simulink model "RF_KC_Time_AxisA4"  (R2020a)
settings: Solver=FixedStepAuto  StartTime=0.0  StopTime=10  FixedStep=0.001  RelTol=1e-3  EnableMultiTasking=on
values from neighbouring files (symbols this model uses):
  A_DC_ESO = [-L1 1 0 0;-L2 0 1 0;-L3 0 0 0;0 0 L4_DCESO/b0 0;]    [Code2.m]
  A_ESO = [-L1 1 0;-L2 0 1;-L3 0 0]    [Code2.m]
  A_ESO2 = [-L1 1 0;-L2 0 1;-L3 0 0]    [Code2.m]
  A_GPIO = [-L1 1 0 0;-L2 0 1 0;-L3 0 0 1; -L4 0 0 0]    [Code2.m]
  b0 = 80    [Code2.m]
  B_DC_ESO = [0 L1;b0 L2;0 L3;0 0]    [Code2.m]
  B_ESO = [0 L1;b0 L2;0 L3]    [Code2.m]
  B_ESO2 = [0 L1;b0 L2;0 L3]    [Code2.m]
  B_GPIO = [0 L1;b0 L2;0 L3;0 L4]    [Code2.m]
  C_DC_ESO = eye(4)    [Code2.m]
  C_ESO = eye(3)    [Code2.m]
  C_ESO2 = eye(3)    [Code2.m]
  C_GPIO = eye(4)    [Code2.m]
  D_DC_ESO = [0 0;0 0;0 0;0 0]    [Code2.m]
  D_ESO = [0 0;0 0;0 0]    [Code2.m]
  D_ESO2 = [0 0;0 0;0 0]    [Code2.m]
  D_GPIO = [0 0;0 0;0 0;0 0]    [Code2.m]
  den_G_invse = den_G_invse{1,1}    [Code2.m]
  den_Q = den_Q{1,1}    [Code2.m]
  num_G_invse = num_G_invse{1,1}    [Code2.m]
  num_Q = num_Q{1,1}    [Code2.m]
  wc = 3*2*pi    (= 18.8495559215)    [Code2.m]
undefined symbols (not defined in the file or in its folder): den_GV, num_GV, taoP
libraries: simulink x1, commnoisgen2 x1
settings Model: Creator=chaosir  LastModifiedBy=Laptop
settings DataIOCC: LimitDataPoints=on  SaveFormat=StructureWithTime  ReturnWorkspaceOutputs=off
settings OptimizationCC: LifeSpan=inf
settings DebuggingCC: SolverPrmCheckMsg=warning  SFUnexpectedBacktrackingDiag=warning  SFNoUnconditionalDefaultTransitionDiag=warning  SFExecutionAtInitializationDiag=none  ArithmeticOperatorsInVariantConditions=warning
settings HardwareCC: ProdBitPerPointer=32  ProdBitPerSizeT=32  ProdBitPerPtrDiffT=32  ProdLargestAtomicFloat=None  ProdIntDivRoundTo=Undefined  ProdEndianess=Unspecified  ProdWordSize=32  ProdHWDeviceType=32-bit Generic
settings ModelReferenceCC: PropagateSignalLabelsOutOfModel=off
settings SFSimCC: SimUseLocalCustomCode=off  CustomCodeUndefinedFunction=UseInterfaceOnly
settings RTWCC: RTWUseLocalCustomCode=off
settings CodeAppCC: StateflowObjectComments=on
settings GRTTargetCC: TargetLangStandard=C89/C90 (ANSI)
settings ConfigComp: CovMetricSettings=dw  CovHtmlReporting=on  CovSaveCumulativeToWorkspaceVar=on  CovSaveSingleToWorkspaceVar=on  CovExternalEMLEnable=off  CovSFcnEnable=off
settings SimscapeCC: SimscapeNormalizeSystem=off
settings ConfigurationSet: Description=SimMechanics 2G

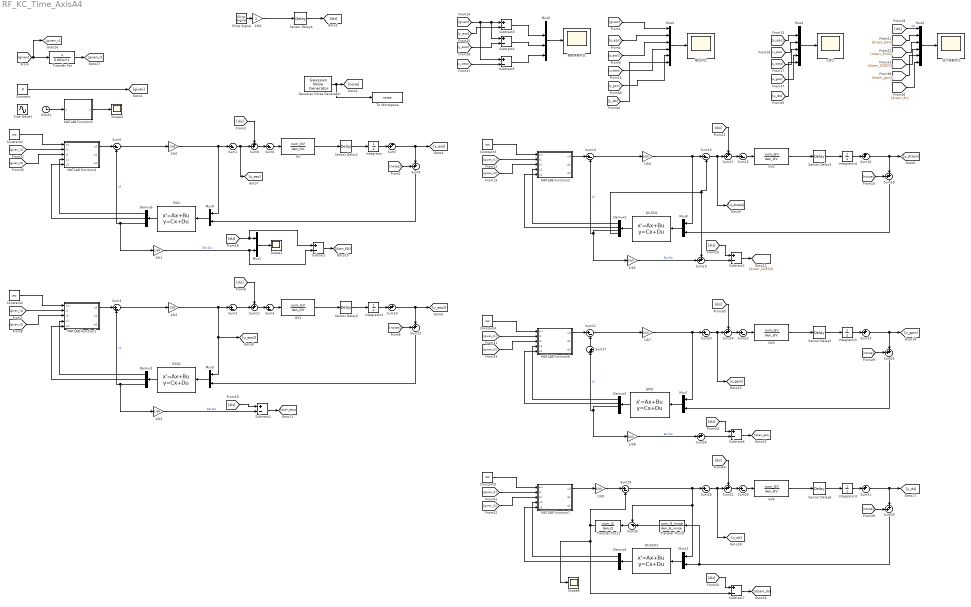
== system RF_KC_Time_AxisA4 ==
  1/b{0..5,7..9} (9 alike) : Gain  Gain=1/b0
  1/b6 : Gain  Gain=2
  Chirp Signal : simulink/Sources/Chirp Signal  f1=0.2  T=7.5  f2=1
  Clock1 : Clock
  Constant : Constant  Value=0
  Constant{1..5} (5 alike) : Constant  Value=wc
  DC-ESO : StateSpace  A=A_DC_ESO  B=B_DC_ESO  C=C_DC_ESO  D=D_DC_ESO
  DC-ESO1 : StateSpace  A=A_ESO  B=B_ESO  C=C_ESO  D=D_ESO
  Demux1 : Demux  Outputs=3
  Demux2 : Demux
  Demux3 : Demux
  Demux4 : Demux  Outputs=3
  Demux5 : Demux  Outputs=3
  ESO : StateSpace  A=A_ESO  B=B_ESO  C=C_ESO  D=D_ESO
  ESO2 : StateSpace  A=A_ESO2  B=B_ESO2  C=C_ESO2  D=D_ESO2
  GPIO : StateSpace  A=A_GPIO  B=B_GPIO  C=C_GPIO  D=D_GPIO
  GV{,1..4} (5 alike) : TransferFcn  Numerator=num_GV  Denominator=den_GV
  Gaussian Noise Generator : commnoisgen2/Gaussian Noise Generator  m=0  d=1e-6  s=0  Ts=0.001  frameBased=off  sampPerFrame=1  orient=off  outDataType=double
      settings: SourceProductBaseCode=CM
  Integrator{,1..4} (5 alike) : Integrator
  MATLAB Function1 : MATLAB Function  TreatAsAtomicUnit=on
  MATLAB Function2 : MATLAB Function  TreatAsAtomicUnit=on
  MATLAB Function4 : MATLAB Function  TreatAsAtomicUnit=on
  MATLAB Function5 : MATLAB Function  TreatAsAtomicUnit=on
  MATLAB Function6 : MATLAB Function  TreatAsAtomicUnit=on
  MATLAB Function7 : MATLAB Function  TreatAsAtomicUnit=on
  Mux{1,5,7..9,11} (6 alike) : Mux  Inputs=2
  Mux2 : Mux  Inputs=6
  Mux3 : Mux  Inputs=6
  Mux4 : Mux  Inputs=6
  Mux6 : Mux
  Scope1 : Scope
  Scope3 : Scope
  Scope6 : Scope
  Sensor Delay{1..3,5..6} (5 alike) : TransportDelay  DelayTime=taoP  PadeOrder=5
  Sensor Delay4 : TransportDelay  DelayTime=3  PadeOrder=5
  Sine Wave1 : Sin  Amplitude=40  Frequency=2*pi*0.08  SampleTime=0
  Subtract{,1..7} (8 alike) : Sum  Inputs=+-
  Sum{1..6,13..15,20..22,28..30} (15 alike) : Sum  Inputs=|+-
  Sum{7..12,16..19,23..26,31..33} (17 alike) : Sum  Inputs=++|
  Sum27 : Sum  Inputs=|++
  Sum35 : Sum  Inputs=-+|
  To Workspace : ToWorkspace  VariableName=noise  SampleTime=-1
  Transfer Fcn : TransferFcn  Numerator=[1 0]  Denominator=[0.001 1]
  Transfer Fcn10 : TransferFcn  Numerator=num_G_invse  Denominator=den_G_invse
  Transfer Fcn11 : TransferFcn  Numerator=num_Q  Denominator=den_Q
  u对比 : Scope
  估计误差对比 : Scope
  跟踪误差对比 : Scope
  输出对比 : Scope
  wires:
  Mux9/1 -> ESO/1
  ESO/1 -> Demux5/1
  Sum1/1 -> [u_eso], Sum8/2
  Mux2/1 -> 输出对比/1
  Sum6/1 -> GV/1
  Demux5/3 -> Sum5/2, 1/b1/1  "z3"
  Sum5/1 -> 1/b0/1
  Sensor Delay1/1 -> Integrator/1
  Sum9/1 -> Mux9/2
  Integrator/1 -> Sum7/2
  Sum8/1 -> Sum6/1
  [noise] -> Sum9/1
  Sum7/1 -> Sum9/2, [y_eso]
  Constant1/1 -> MATLAB Function4/1(wc)
  Transfer Fcn/1 -> [given_r2]
  Demux5/1 -> MATLAB Function4/4(x1)
  [given] -> [given_r1], Transfer Fcn/1
  [given_r2] -> MATLAB Function4/3(r2)
  [given_r1] -> MATLAB Function4/2(r1)
  [given] -> Mux2/1
  Demux5/2 -> MATLAB Function4/5(x2)
  1/b0/1 -> Sum1/1, Mux9/1
  Mux1/1 -> Scope1/1
  1/b1/1 -> Subtract/2, Mux1/2  "Est Dis"
  GV/1 -> Sensor Delay1/1
  MATLAB Function4/1(u0) -> Sum5/1
  Gaussian Noise Generator/1 -> To Workspace/1, [noise]
  [noise] -> Sum12/1
  1/b3/1 -> Subtract1/2  "Est Dis"
  Demux1/2 -> MATLAB Function1/5(x2)
  Sum12/1 -> Mux5/2
  Constant2/1 -> MATLAB Function1/1(wc)
  Sum10/1 -> [y_eso2], Sum12/2
  1/b2/1 -> Sum2/1, [u_eso2], Mux5/1
  Sum11/1 -> Sum4/1
  [given_r2] -> MATLAB Function1/3(r2)
  [given_r1] -> MATLAB Function1/2(r1)
  Sum3/1 -> 1/b2/1
  Sum4/1 -> GV1/1
  Demux1/1 -> MATLAB Function1/4(x1)
  GV1/1 -> Sensor Delay2/1
  Integrator2/1 -> Sum10/2
  Sum2/1 -> Sum11/2
  Demux1/3 -> 1/b3/1, Sum3/2  "z3"
  ESO2/1 -> Demux1/1
  MATLAB Function1/1(u0) -> Sum3/1
  Sensor Delay2/1 -> Integrator2/1
  Mux5/1 -> ESO2/1
  [dis] -> Sum17/1
  Demux2/4 -> Sum13/2, Sum19/1
  [noise] -> Sum18/1
  Demux2/2 -> MATLAB Function2/5(x2)
  Sum18/1 -> Mux8/2
  Constant3/1 -> MATLAB Function2/1(wc)
  Sum16/1 -> Sum18/2, [y_dceso]
  1/b4/1 -> Sum13/1, Mux8/1
  Sum17/1 -> Sum15/1
  [given_r2] -> MATLAB Function2/3(r2)
  [given_r1] -> MATLAB Function2/2(r1)
  Sum14/1 -> 1/b4/1
  Sum15/1 -> GV2/1
  Demux2/1 -> MATLAB Function2/4(x1)
  GV2/1 -> Sensor Delay3/1
  Integrator4/1 -> Sum16/2
  Sum13/1 -> [u_dceso], Sum17/2
  Demux2/3 -> 1/b5/1, Sum14/2  "z3"
  DC-ESO/1 -> Demux2/1
  MATLAB Function2/1(u0) -> Sum14/1
  Sensor Delay3/1 -> Integrator4/1
  Mux8/1 -> DC-ESO/1
  [y_eso] -> Mux2/2
  [y_eso2] -> Mux2/3
  [y_dceso] -> Mux2/4
  Mux4/1 -> u对比/1
  [u_eso] -> Mux4/2
  [u_eso2] -> Mux4/3
  [u_dceso] -> Mux4/4
  [dis] -> Sum8/1
  [dis] -> Sum11/1
  [dis] -> Subtract/1, Mux1/1
  Subtract/1 -> [diserr_ESO]
  Subtract1/1 -> [diserr_ESO2]
  [dis] -> Subtract1/1
  1/b5/1 -> Sum19/2  "Est Dis"
  Subtract2/1 -> [diserr_DCESO]
  Sum19/1 -> Subtract2/2
  [dis] -> Subtract2/1
  [diserr_DCESO] -> Mux3/4
  [diserr_ESO2] -> Mux3/3
  [diserr_ESO] -> Mux3/2
  Mux3/1 -> 估计误差对比/1
  Clock1/1 -> MATLAB Function5/1(t)
  MATLAB Function5/1(y) -> Scope3/1
  [given] -> Subtract5/1, Subtract4/1, Subtract3/1
  [y_eso] -> Subtract3/2
  [y_eso2] -> Subtract4/2
  [y_dceso] -> Subtract5/2
  Mux6/1 -> 跟踪误差对比/1
  Subtract3/1 -> Mux6/2
  Subtract4/1 -> Mux6/3
  Subtract5/1 -> Mux6/4
  Constant/1 -> [given]
  [dis] -> Mux3/1  "dis"
  [noise] -> Sum25/1
  Sum26/1 -> Subtract6/2
  1/b8/1 -> Sum26/2  "Est Dis"
  Mux7/1 -> GPIO/1
  Sum22/1 -> GV3/1
  Demux3/1 -> MATLAB Function6/4(x1)
  Subtract6/1 -> [diserr_gpio]
  Sensor Delay5/1 -> Integrator1/1
  MATLAB Function6/1(u0) -> Sum21/1
  Constant4/1 -> MATLAB Function6/1(wc)
  Sum21/1 -> 1/b7/1
  Demux3/3 -> 1/b8/1, Sum27/1  "z3"
  [dis] -> Subtract6/1
  Sum23/1 -> Sum25/2, [y_gpio]
  GPIO/1 -> Demux3/1
  Sum20/1 -> [u_gpio], Sum24/2
  Integrator1/1 -> Sum23/2
  GV3/1 -> Sensor Delay5/1
  Sum24/1 -> Sum22/1
  Demux3/2 -> MATLAB Function6/5(x2)
  [given_r1] -> MATLAB Function6/2(r1)
  [dis] -> Sum24/1
  [given_r2] -> MATLAB Function6/3(r2)
  Sum25/1 -> Mux7/2
  1/b7/1 -> Sum20/1, Mux7/1
  Sum27/1 -> Sum21/2
  [y_gpio] -> Mux2/5
  [diserr_gpio] -> Mux3/5
  Sum32/1 -> Sum30/1
  Demux4/2 -> MATLAB Function7/5(x2)
  [dis] -> Sum32/1
  [given_r1] -> MATLAB Function7/2(r1)
  Integrator3/1 -> Sum31/2
  Sum28/1 -> [u_do], Sum32/2
  Sum31/1 -> Sum33/2, [y_do]
  [dis] -> Subtract7/1
  GV4/1 -> Sensor Delay6/1
  Demux4/1 -> MATLAB Function7/4(x1)
  Sensor Delay6/1 -> Integrator3/1
  Transfer Fcn11/1 -> Sum29/2, Scope6/1, Subtract7/2
  Sum30/1 -> GV4/1
  MATLAB Function7/1(u0) -> 1/b9/1
  Constant5/1 -> MATLAB Function7/1(wc)
  [noise] -> Sum33/1
  Subtract7/1 -> [diserr_do]
  Sum33/1 -> Transfer Fcn10/1, Mux11/2
  [given_r2] -> MATLAB Function7/3(r2)
  DC-ESO1/1 -> Demux4/1
  Transfer Fcn10/1 -> Sum35/2
  Sum35/1 -> Transfer Fcn11/1
  Sum29/1 -> Sum28/1, Sum35/1, Mux11/1
  [y_do] -> Mux2/6
  [u_do] -> Mux4/6
  [diserr_do] -> Mux3/6
  1/b9/1 -> Sum29/1
  Mux11/1 -> DC-ESO1/1
  Chirp Signal/1 -> 1/b6/1
  1/b6/1 -> Sensor Delay4/1
  [u_gpio] -> Mux4/5
  Sensor Delay4/1 -> [dis]

== matlab function RF_KC_Time_AxisA4/MATLAB Function1 ==
  data: wc input; r1 input; u0 output; r2 input; x1 input; x2 input; e1 output; e2 output
function [u0,e1,e2] = feedback_law(wc,r1,r2,x1,x2)

    k1 = wc^2;
    k2 = 2*wc;
    e1 = (r1-x1);
    e2 = (r2-x2);
    u0 = k1*e1+k2*e2;
    
end

== matlab function RF_KC_Time_AxisA4/MATLAB Function2 ==
  data: wc input; r1 input; u0 output; r2 input; x1 input; x2 input; e1 output; e2 output
function [u0,e1,e2] = feedback_law(wc,r1,r2,x1,x2)

    k1 = wc^2;
    k2 = 2*wc;
    e1 = (r1-x1);
    e2 = (r2-x2);
    u0 = k1*e1+k2*e2;
    
end

== matlab function RF_KC_Time_AxisA4/MATLAB Function5 ==
  data: t input; y output
function y = fcn(t)

    y1 = 0;
    y2 = -3;
    y3 = 4;
    t1 = 2;
    t2 = 5;
    if t < t1
        y = y1;
    elseif t >= t1 && t < t1 + 1
        % 使用平滑的非线性过渡函数，这里用三次函数过渡
        alpha = (t - t1)/1;
        y = y1 + (y2 - y1)*alpha^3*(10 - 15*alpha + 6*alpha^2);
    elseif t >= t1 + 1 && t < t2
        y = y2;
    elseif t >= t2 && t < t2 + 1
        % 再次使用平滑的非线性过渡函数
        alpha = (t - t2)/1;
        y = y2 + (y3 - y2)*alpha^3*(10 - 15*alpha + 6*alpha^2);
    else
        y = y3;
    end
    
end

== matlab function RF_KC_Time_AxisA4/MATLAB Function4 ==
  data: wc input; r1 input; u0 output; r2 input; x1 input; x2 input; e1 output; e2 output
function [u0,e1,e2] = feedback_law(wc,r1,r2,x1,x2)

    k1 = wc^2;
    k2 = 2*wc;
    e1 = (r1-x1);
    e2 = (r2-x2);
    u0 = k1*e1+k2*e2;
    
end

== matlab function RF_KC_Time_AxisA4/MATLAB Function6 ==
  data: wc input; r1 input; u0 output; r2 input; x1 input; x2 input; e1 output; e2 output
function [u0,e1,e2] = feedback_law(wc,r1,r2,x1,x2)

    k1 = wc^2;
    k2 = 2*wc;
    e1 = (r1-x1);
    e2 = (r2-x2);
    u0 = k1*e1+k2*e2;
    
end

== matlab function RF_KC_Time_AxisA4/MATLAB Function7 ==
  data: wc input; r1 input; u0 output; r2 input; x1 input; x2 input; e1 output; e2 output
function [u0,e1,e2] = feedback_law(wc,r1,r2,x1,x2)

    k1 = wc^2;
    k2 = 2*wc;
    e1 = (r1-x1);
    e2 = (r2-x2);
    u0 = k1*e1+k2*e2;
    
end
